simulink model "spring_mass_damper"  (R2016a)
settings: Solver=VariableStepAuto  SolverMode=SingleTasking  StartTime=0.0  StopTime=10.0  RelTol=1e-3
libraries: fl_lib x6, nesl_utility x3
settings Model: Creator=AkashG_v13  LastModifiedBy=Tanay
settings DebuggingCC: SFUnexpectedBacktrackingDiag=error  SFNoUnconditionalDefaultTransitionDiag=error
settings GRTTargetCC: TargetLangStandard=C99 (ISO)  GeneratePreprocessorConditionals=Use local settings
settings ConfigComp: CovMetricSettings=dwe  CovHtmlReporting=off  CovSaveCumulativeToWorkspaceVar=off  CovSaveSingleToWorkspaceVar=off  CovExternalEMLEnable=on

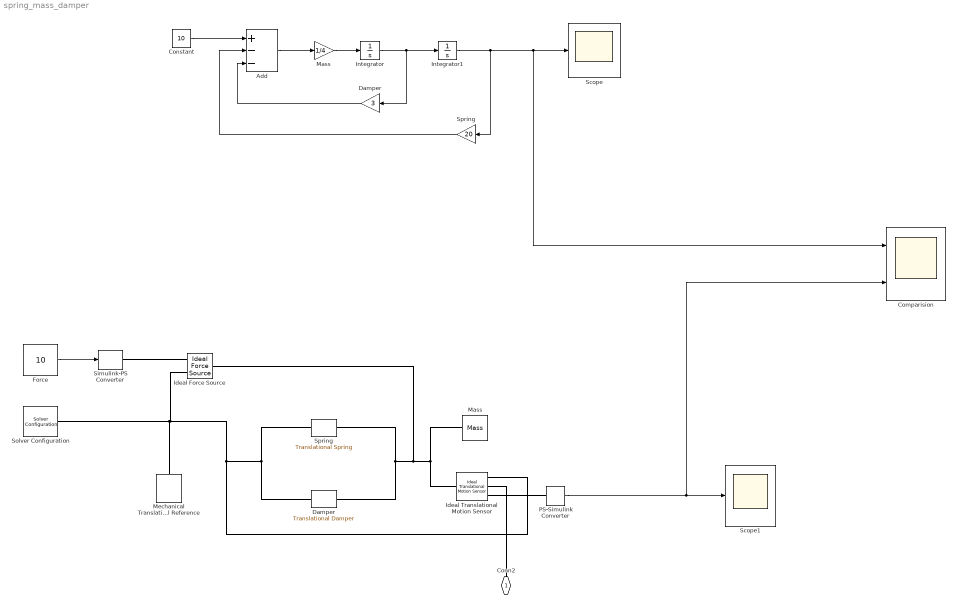
== system spring_mass_damper ==
  " Damper" : fl_lib/Mechanical/Translational Elements/Translational Damper  D=3 N/(m/s)  v_specify=off  v_priority=None  v=0 m/s  f_specify=off  f_priority=None  f=0 N
  " Spring" : fl_lib/Mechanical/Translational Elements/Translational Spring  spr_rate=20 N/m  v_specify=off  v_priority=None  v=0 m/s  f_specify=off  f_priority=None  f=0 N  x_specify=off  x_priority=High  x=0 m
  Add : Sum  Inputs=+--
  Comparision : Scope  NumInputPorts=2
  Constant : Constant  Value=10
  Damper : Gain  Gain=3
  Force : Constant  Value=10
  Ideal Force Source : fl_lib/Mechanical/Mechanical Sources/Ideal Force Source
  Ideal Translational Motion Sensor : fl_lib/Mechanical/Mechanical Sensors/Ideal Translational Motion Sensor  offset=0 m
  Integrator : Integrator
  Integrator1 : Integrator
  "Mass " : Gain  Gain=1/4
  "Mass " : fl_lib/Mechanical/Translational Elements/Mass  mass=4 kg  v_specify=off  v_priority=High  v=0 m/s  f_specify=off  f_priority=None  f=0 N
  Mechanical Translational Reference : fl_lib/Mechanical/Translational Elements/Mechanical Translational Reference
  PS-Simulink Converter : nesl_utility/PS-Simulink Converter  PhysicalDomain=network_engine_domain  SubClassName=ps_output  LeftPortType=input  RightPortType=output  PseudoPeriodic=off  Frequencies=[]  Unit=1  AffineConversion=off
  Scope : Scope
  Scope1 : Scope
  Simulink-PS Converter : nesl_utility/Simulink-PS Converter  PhysicalDomain=network_engine_domain  SubClassName=ps_input  LeftPortType=input  RightPortType=output  PseudoPeriodic=off  Frequencies=[]  NoiseDistribution=none  NoiseParameters=[]  Unit=1  AffineConversion=off  InputFiltering=off  SimscapeFilterOrder=1  InputFilterTimeConstant=0.001  UdotUserProvided=1
  Solver Configuration : nesl_utility/Solver Configuration  PhysicalDomain=network_engine_domain  SubClassName=solver  LeftPortType=input  RightPortType=generic  Accelerate=off  Tones=[]  Harmonics=[]  SimulateNoise=off  Profile=off  UseLocalSampling=off  EnableSwitchedLinearOptims=on  FrequencyDomain=off  UseCCode=off  RelTol=0.001  AbsTol=1e-06  MinStep=1e-09  ToWorkspace=off  RevertToSquareIcSolve=off  NumHomotopyIterations=100  PhasorMode=off  PhasorModeNumHarmonics=1  OverrideAbsTol=off  DoDC=off  ResidualTolerance=1e-09  UseLocalSolver=off  LocalSolverChoice=NE_BACKWARD_EULER_ADVANCER  LocalSolverSampleTime=0.001  DoFixedCost=off  MaxNonlinIter=3  MaxModeIter=2  LinearAlgebra=Sparse  DelaysMemoryBudget=1024  AutomaticFiltering=on  FilteringTimeConstant=0.001
  Spring : Gain  Gain=20
  Conn2 : PMIOPort  Port=1  Side=Right
  wires:
  Spring/1 -> Add/2
  Damper/1 -> Add/3
  Add/1 -> "Mass "/1
  Constant/1 -> Add/1
  Integrator/1 -> Damper/1, Integrator1/1
  "Mass "/1 -> Integrator/1
  Integrator1/1 -> Comparision/1, Scope/1, Spring/1
  Force/1 -> Simulink-PS Converter/1
  PS-Simulink Converter/1 -> Comparision/2, Scope1/1
  connections:
  " Spring"/RConn1 -- Ideal Force Source/LConn1 -- "Mass "/LConn1 -- Ideal Translational Motion Sensor/LConn1 -- " Damper"/RConn1
  " Damper"/LConn1 -- " Spring"/LConn1 -- Ideal Translational Motion Sensor/RConn1 -- Solver Configuration/RConn1 -- Mechanical Translational Reference/LConn1 -- Ideal Force Source/RConn2
  Ideal Translational Motion Sensor/RConn3 -- PS-Simulink Converter/LConn1
  Simulink-PS Converter/RConn1 -- Ideal Force Source/RConn1
  Ideal Translational Motion Sensor/RConn2 -- Conn2/RConn1
